simulink model "droneENGK38"  (R2018b)
settings: Solver=VariableStepAuto  StartTime=0.0  StopTime=12  RelTol=1e-3
values from neighbouring files (symbols this model uses):
  Cx = 0.3    [dadosProj_Drone.m]
  Cy = 0.1    [dadosProj_Drone.m]
  fimax = 0.26    [dadosProj_Drone.m]
  g = 9.8    [dadosProj_Drone.m]
  Kpsi = 1    [dadosProj_Drone.m]
  Kz = 1.3    [dadosProj_Drone.m]
  psimax = 1.74    [dadosProj_Drone.m]
  thetamax = 0.26    [dadosProj_Drone.m]
  tpsi = 0.3    [dadosProj_Drone.m]
  tz = 0.4    [dadosProj_Drone.m]
  wfi = 4.47    [dadosProj_Drone.m]
  wtheta = 4.47    [dadosProj_Drone.m]
  zetafi = 0.5    [dadosProj_Drone.m]
  zetatheta = 0.5    [dadosProj_Drone.m]
  zmax = 1.0    (= 1)    [dadosProj_Drone.m]
settings Model: Creator=root  LastModifiedBy=root

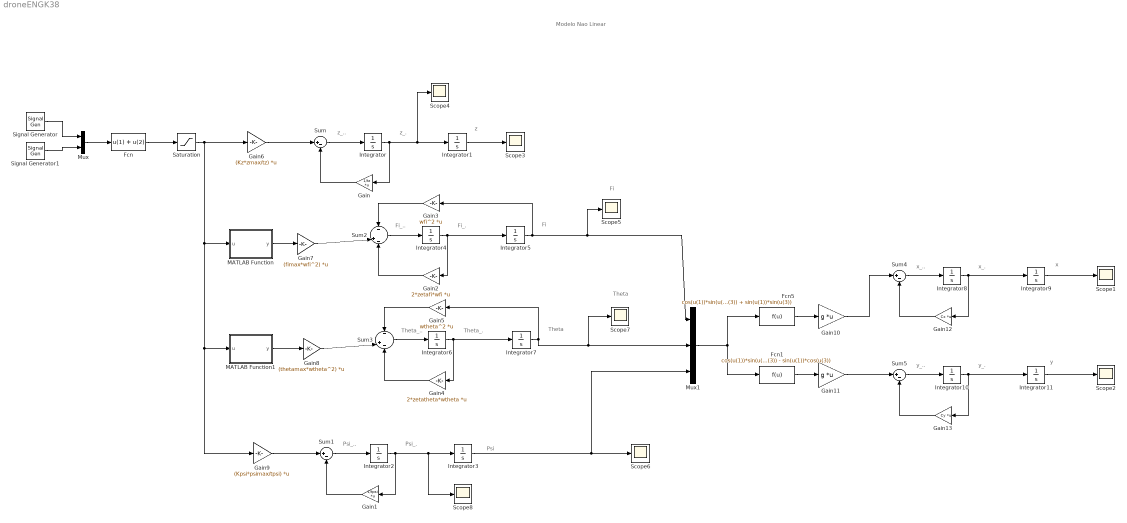
== system droneENGK38 ==
  note: Modelo Nao Linear
  note: z_..
  note: z
  note: z_.
  note: Psi
  note: Psi_.
  note: Psi_..
  note: Fi
  note: Fi_.
  note: Fi_..
  note: Theta_..
  note: Theta_.
  note: Theta
  note: x
  note: x_.
  note: x_..
  note: y
  note: y_.
  note: y_..
  note: Fi
  note: Theta
  Fcn : Fcn  Expr=u(1) + u(2)
  Fcn1 : Fcn  Expr=cos(u(1))*sin(u(2))*sin(u(3)) - sin(u(1))*cos(u(3))
  Fcn5 : Fcn  Expr=cos(u(1))*sin(u(2))*cos(u(3)) + sin(u(1))*sin(u(3))
  Gain : Gain  Gain=1/tz  Multiplication=Matrix(K*u)
  Gain1 : Gain  Gain=1/tpsi  Multiplication=Matrix(K*u)
  Gain10 : Gain  Gain=g  Multiplication=Matrix(K*u)
  Gain11 : Gain  Gain=g  Multiplication=Matrix(K*u)
  Gain12 : Gain  Gain=Cx  Multiplication=Matrix(K*u)
  Gain13 : Gain  Gain=Cy  Multiplication=Matrix(K*u)
  Gain2 : Gain  Gain=2*zetafi*wfi  Multiplication=Matrix(K*u)
  Gain3 : Gain  Gain=wfi^2  Multiplication=Matrix(K*u)
  Gain4 : Gain  Gain=2*zetatheta*wtheta  Multiplication=Matrix(K*u)
  Gain5 : Gain  Gain=wtheta^2  Multiplication=Matrix(K*u)
  Gain6 : Gain  Gain=(Kz*zmax/tz)  Multiplication=Matrix(K*u)
  Gain7 : Gain  Gain=(fimax*wfi^2)  Multiplication=Matrix(K*u)
  Gain8 : Gain  Gain=(thetamax*wtheta^2)  Multiplication=Matrix(K*u)
  Gain9 : Gain  Gain=(Kpsi*psimax/tpsi)  Multiplication=Matrix(K*u)
  Integrator{,1..11} (12 alike) : Integrator
  MATLAB Function : MATLAB Function  TreatAsAtomicUnit=on
  MATLAB Function1 : MATLAB Function  TreatAsAtomicUnit=on
  Mux : Mux  Inputs=2
  Mux1 : Mux  Inputs=3
  Saturation : Saturate  UpperLimit=1  LowerLimit=-1
  Scope{1..8} (8 alike) : Scope
  Signal Generator : SignalGenerator  Amplitude=0.5  Frequency=(2*pi)/5  Units=rad/sec
  Signal Generator1 : SignalGenerator  Amplitude=0.3  Frequency=(2*pi)/(0.2*5)  Units=rad/sec
  Sum{,1,4..5} (4 alike) : Sum  Inputs=|+-
  Sum2 : Sum  Inputs=-|+-
  Sum3 : Sum  Inputs=-|+-
  wires:
  Mux/1 -> Fcn/1
  Signal Generator/1 -> Mux/1
  Signal Generator1/1 -> Mux/2
  Fcn/1 -> Saturation/1
  Saturation/1 -> Gain6/1, MATLAB Function/1(u), Gain9/1, MATLAB Function1/1(u)
  Gain6/1 -> Sum/1
  Sum/1 -> Integrator/1
  Gain/1 -> Sum/2
  Integrator/1 -> Scope4/1, Integrator1/1, Gain/1
  Integrator2/1 -> Scope8/1, Integrator3/1, Gain1/1
  Sum1/1 -> Integrator2/1
  Gain9/1 -> Sum1/1
  Gain1/1 -> Sum1/2
  Integrator4/1 -> Integrator5/1, Gain2/1
  Sum2/1 -> Integrator4/1
  MATLAB Function/1(y) -> Gain7/1
  Gain7/1 -> Sum2/2
  Gain2/1 -> Sum2/3
  Gain3/1 -> Sum2/1
  Integrator7/1 -> Scope7/1, Mux1/2, Gain5/1
  Gain8/1 -> Sum3/2
  Gain5/1 -> Sum3/1
  Gain4/1 -> Sum3/3
  Integrator6/1 -> Integrator7/1, Gain4/1
  Sum3/1 -> Integrator6/1
  MATLAB Function1/1(y) -> Gain8/1
  Integrator5/1 -> Scope5/1, Mux1/1, Gain3/1
  Integrator3/1 -> Mux1/3, Scope6/1
  Mux1/1 -> Fcn1/1, Fcn5/1
  Fcn5/1 -> Gain10/1
  Fcn1/1 -> Gain11/1
  Sum4/1 -> Integrator8/1
  Integrator8/1 -> Integrator9/1, Gain12/1
  Gain10/1 -> Sum4/1
  Gain12/1 -> Sum4/2
  Sum5/1 -> Integrator10/1
  Integrator10/1 -> Integrator11/1, Gain13/1
  Gain11/1 -> Sum5/1
  Gain13/1 -> Sum5/2
  Integrator11/1 -> Scope2/1
  Integrator9/1 -> Scope1/1
  Integrator1/1 -> Scope3/1

== matlab function droneENGK38/MATLAB Function1 ==
  data: u input; y output
% ==> Funcao para calcular valor de K_fi
function y = k_theta(u)
    k_theta_min = 1;
    k_theta_max = 2;
    
    if abs(u) > 0.5
        u = k_theta_min*u;
    else       
        u = k_theta_max*u;
    end
y = u;

== matlab function droneENGK38/MATLAB Function ==
  data: u input; y output
% ==> Funcao para calcular valor de K_fi
function y = k_fi(u)
    k_fi_min = 1;
    k_fi_max = 2;
    
    if abs(u) > 0.5
        u = k_fi_min*u;
    else       
        u = k_fi_max*u;
    end
y = u;
